simulink model "MSC_MATLAB_AGV_ROMB_diploma_3pcs_final"  (R2016b)
settings: Solver=VariableStepAuto  StartTime=0.0  StopTime=100  RelTol=1e-3
PreLoadFcn:
  | load('C:\Users\CAD_Admin\AGV\gostask\warehouse1.mat')
  | AGV_Simple_ New
values from neighbouring files (symbols this model uses):
  AGVs =     [algorithm_test.mat]
  contr1_kp = 0.4    [algorithm_test.mat]
  LF_AngVel = 30    [algorithm_test.mat]
  lns = lns1    [CMDTrackRead.m]    (also in algorithm_test.mat = [1 3 5 7 9 11 13 15 17 19 21 23 ... (242 elements, 121x2)]; warehouseGubkina.mat = [9 3 2 10 4 8 7 3 8 5 7 6 ... (26 elements, 13x2)]; warehouseGubkinaNew.mat = [9 15 17 10 19 11 13 3 3 5 5 8 ... (46 elements, 23x2)])
  pnts = RoundingPnts(pnts)    [Avoidance_Testing.m]    (also in CMDTrackRead.m = pnts1; algorithm_test.mat = [-350 450 0 0 100 100 -340 -260 -100 -100 -350 450 ... (321 ; warehouseGubkina.mat = [4100 4100 4100 3646 3646 3646 3822 3822 4100 4198.5 3822 34; warehouseGubkinaNew.mat = [4100 4100 4100 3646 3646 3646 3822 3822 4100 4198.5 3822 38)
  SteeringVel = 10    [algorithm_test.mat]
  T_Motor = 0.05    [algorithm_test.mat]
  tau_DiscreteSensor = 0.3    [algorithm_test.mat]
  tau_Motor = 0.125    [algorithm_test.mat]
  value0 = [23350 22900 22450 20300 17050 13100 10500 8700 8100 7800 7700 7800 ... (21 elements, 21x1)]    [algorithm_test.mat]
  x0 = 10    [SecondAGV.m]    (also in algorithm_test.mat = [-70 -50 -40 -35 -30 -25 -20 -15 -10 -5 0 5 ... (21 elements)
undefined symbols (not defined in the file): ADAMS_cwd, ADAMS_exec, ADAMS_host, ADAMS_init, ADAMS_inputs, ADAMS_outputs, ADAMS_prefix, ADAMS_static, ADAMS_sysdir
libraries: simulink x21
(part 2 of 2)

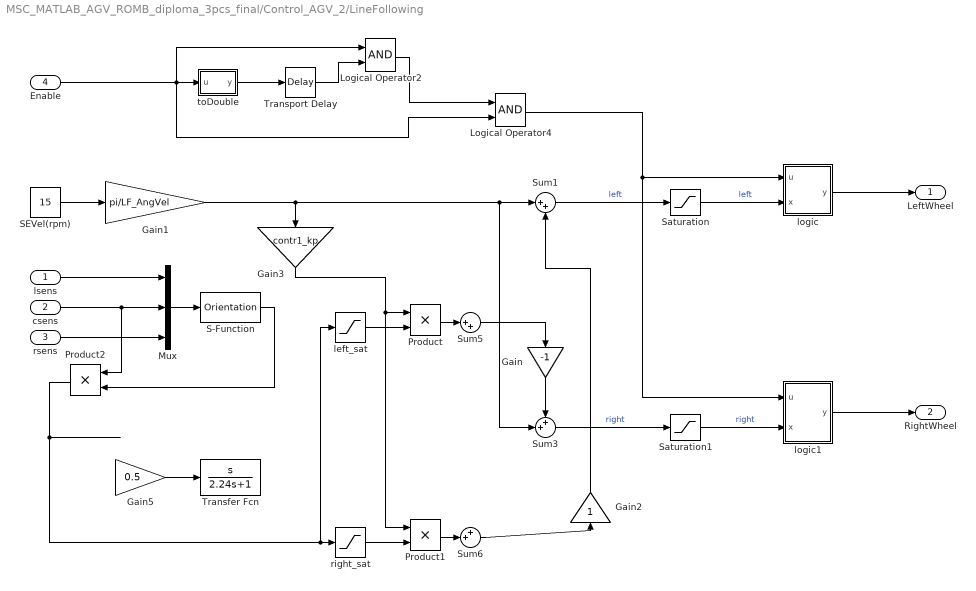
== system MSC_MATLAB_AGV_ROMB_diploma_3pcs_final/Control_AGV_2/LineFollowing ==
  lsens : Inport
  csens : Inport  Port=2
  rsens : Inport  Port=3
  Enable : Inport  Port=4
  Gain : Gain  Gain=-1
  Gain1 : Gain  Gain=pi/LF_AngVel
  Gain2 : Gain
  Gain3 : Gain  Gain=contr1_kp
  Gain5 : Gain  Gain=0.5
  Logical Operator2 : Logic  AllPortsSameDT=off  OutDataTypeStr=boolean
  Logical Operator4 : Logic  AllPortsSameDT=off  OutDataTypeStr=boolean
  Mux : Mux  Inputs=3
  Product : Product
  Product1 : Product
  Product2 : Product
  S-Function : S-Function  FunctionName=Orientation  SFunctionDeploymentMode=off  EnableBusSupport=off
  SEVel(rpm) : Constant  Value=15
  Saturation : Saturate  UpperLimit=inf  LowerLimit=0
  Saturation1 : Saturate  UpperLimit=inf  LowerLimit=0
  Sum1 : Sum  Inputs=|++
  Sum3 : Sum  Inputs=++|
  Sum5 : Sum  Inputs=|++
  Sum6 : Sum  Inputs=++|
  Transfer Fcn : TransferFcn  Numerator=[1 0]  Denominator=[2.24 1]
  Transport Delay : TransportDelay  DelayTime=0.05
  left_sat : Saturate  UpperLimit=0  LowerLimit=-10
  logic : MATLAB Function  TreatAsAtomicUnit=on
  logic1 : MATLAB Function  TreatAsAtomicUnit=on
  right_sat : Saturate  UpperLimit=10  LowerLimit=0
  toDouble : MATLAB Function  TreatAsAtomicUnit=on
  LeftWheel : Outport
  RightWheel : Outport  Port=2
  wires:
  SEVel(rpm)/1 -> Gain1/1
  Gain1/1 -> Sum3/2, Sum1/1, Gain3/1
  lsens/1 -> Mux/1
  rsens/1 -> Mux/3
  Sum6/1 -> Gain2/1
  S-Function/1 -> Product2/2
  csens/1 -> Product2/1, Mux/2
  Product2/1 -> left_sat/1, right_sat/1
  Saturation/1 -> logic/2(x)  "left"
  logic/1(y) -> LeftWheel/1
  Saturation1/1 -> logic1/2(x)  "right"
  logic1/1(y) -> RightWheel/1
  Logical Operator2/1 -> Logical Operator4/1
  Enable/1 -> Logical Operator2/1, toDouble/1(u), Logical Operator4/2
  toDouble/1(y) -> Transport Delay/1
  Transport Delay/1 -> Logical Operator2/2
  Logical Operator4/1 -> logic1/1(u), logic/1(u)
  Mux/1 -> S-Function/1
  Gain/1 -> Sum3/1
  Gain2/1 -> Sum1/2
  Sum5/1 -> Gain/1
  Gain3/1 -> Product1/1, Product/1
  right_sat/1 -> Product1/2
  left_sat/1 -> Product/2
  Gain5/1 -> Transfer Fcn/1
  ? -> Sum6/1, Sum5/2
  Product/1 -> Sum5/1
  Product1/1 -> Sum6/2
  Sum3/1 -> Saturation1/1  "right"
  Sum1/1 -> Saturation/1  "left"

== system MSC_MATLAB_AGV_ROMB_diploma_3pcs_final/Control_AGV_2/Steering ==
  lsens : Inport
  csens : Inport  Port=2
  rsens : Inport  Port=3
  Steering : Inport  Port=4
  Enable : Inport  Port=5
  Demux : Demux  Outputs=2
  Gain1 : Gain  Gain=pi/LF_AngVel
  Logical Operator2 : Logic  AllPortsSameDT=off  OutDataTypeStr=boolean
  Logical Operator4 : Logic  AllPortsSameDT=off  OutDataTypeStr=boolean
  Mux : Mux
  Product : Product
  Product2 : Product
  S-Function : S-Function  FunctionName=CartSteering_1  Parameters=lns,pnts  SFunctionDeploymentMode=off  EnableBusSupport=off
  SEVel(rpm) : Constant  Value=SteeringVel
  Saturation : Saturate  UpperLimit=inf  LowerLimit=-inf
  Saturation1 : Saturate  UpperLimit=inf  LowerLimit=-inf
  Transport Delay : TransportDelay  DelayTime=0.2
  left_sat : Saturate  UpperLimit=2  LowerLimit=-2
  logic : MATLAB Function  TreatAsAtomicUnit=on
  logic1 : MATLAB Function  TreatAsAtomicUnit=on
  right_sat : Saturate  UpperLimit=2  LowerLimit=-2
  toDouble : MATLAB Function  TreatAsAtomicUnit=on
  LeftWheel : Outport
  RightWheel : Outport  Port=2
  wires:
  rsens/1 -> Mux/3
  csens/1 -> Mux/2
  lsens/1 -> Mux/1
  Steering/1 -> Mux/4
  Product/1 -> Saturation/1  "left"
  SEVel(rpm)/1 -> Gain1/1
  Product2/1 -> Saturation1/1  "right"
  Gain1/1 -> Product2/1, Product/1
  Saturation/1 -> logic/2(x)  "left"
  Saturation1/1 -> logic1/2(x)  "right"
  Demux/1 -> left_sat/1
  Demux/2 -> right_sat/1
  Mux/1 -> S-Function/1
  S-Function/1 -> Demux/1
  left_sat/1 -> Product/2
  right_sat/1 -> Product2/2
  logic/1(y) -> LeftWheel/1
  logic1/1(y) -> RightWheel/1
  Logical Operator4/1 -> logic1/1(u), logic/1(u)
  Logical Operator2/1 -> Logical Operator4/1
  Enable/1 -> toDouble/1(u), Logical Operator4/2, Logical Operator2/1
  toDouble/1(y) -> Transport Delay/1
  Transport Delay/1 -> Logical Operator2/2

== system MSC_MATLAB_AGV_ROMB_diploma_3pcs_final/Control_AGV_2/Subsystem ==
  Enable : Inport
  LeftWheel : Inport  Port=2
  RightWheel : Inport  Port=3
  Logical Operator2 : Logic  AllPortsSameDT=off  OutDataTypeStr=boolean
  Logical Operator4 : Logic  AllPortsSameDT=off  OutDataTypeStr=boolean
  Transport Delay1 : TransportDelay  DelayTime=0.05
  logic : MATLAB Function  TreatAsAtomicUnit=on
  logic1 : MATLAB Function  TreatAsAtomicUnit=on
  toDouble5 : MATLAB Function  TreatAsAtomicUnit=on
  LeftVel : Outport
  RightVel : Outport  Port=2
  wires:
  Logical Operator2/1 -> Logical Operator4/1
  Enable/1 -> Logical Operator2/1, toDouble5/1(u), Logical Operator4/2
  toDouble5/1(y) -> Transport Delay1/1
  Transport Delay1/1 -> Logical Operator2/2
  Logical Operator4/1 -> logic1/1(u), logic/1(u)
  logic/1(y) -> LeftVel/1
  logic1/1(y) -> RightVel/1
  LeftWheel/1 -> logic/2(x)
  RightWheel/1 -> logic1/2(x)

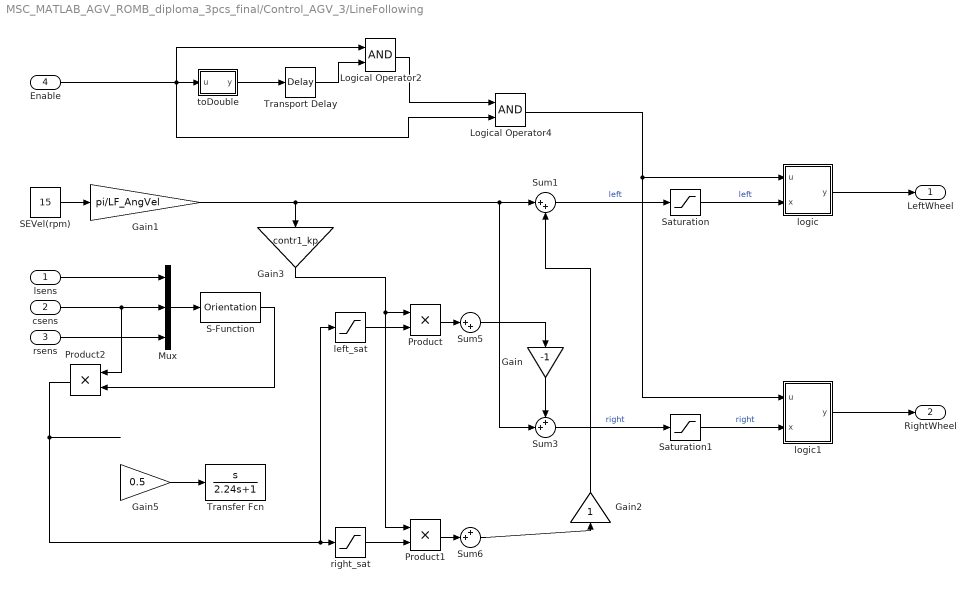
== system MSC_MATLAB_AGV_ROMB_diploma_3pcs_final/Control_AGV_3/LineFollowing ==
  lsens : Inport
  csens : Inport  Port=2
  rsens : Inport  Port=3
  Enable : Inport  Port=4
  Gain : Gain  Gain=-1
  Gain1 : Gain  Gain=pi/LF_AngVel
  Gain2 : Gain
  Gain3 : Gain  Gain=contr1_kp
  Gain5 : Gain  Gain=0.5
  Logical Operator2 : Logic  AllPortsSameDT=off  OutDataTypeStr=boolean
  Logical Operator4 : Logic  AllPortsSameDT=off  OutDataTypeStr=boolean
  Mux : Mux  Inputs=3
  Product : Product
  Product1 : Product
  Product2 : Product
  S-Function : S-Function  FunctionName=Orientation  SFunctionDeploymentMode=off  EnableBusSupport=off
  SEVel(rpm) : Constant  Value=15
  Saturation : Saturate  UpperLimit=inf  LowerLimit=0
  Saturation1 : Saturate  UpperLimit=inf  LowerLimit=0
  Sum1 : Sum  Inputs=|++
  Sum3 : Sum  Inputs=++|
  Sum5 : Sum  Inputs=|++
  Sum6 : Sum  Inputs=++|
  Transfer Fcn : TransferFcn  Numerator=[1 0]  Denominator=[2.24 1]
  Transport Delay : TransportDelay  DelayTime=0.05
  left_sat : Saturate  UpperLimit=0  LowerLimit=-10
  logic : MATLAB Function  TreatAsAtomicUnit=on
  logic1 : MATLAB Function  TreatAsAtomicUnit=on
  right_sat : Saturate  UpperLimit=10  LowerLimit=0
  toDouble : MATLAB Function  TreatAsAtomicUnit=on
  LeftWheel : Outport
  RightWheel : Outport  Port=2
  wires:
  SEVel(rpm)/1 -> Gain1/1
  Gain1/1 -> Sum3/2, Sum1/1, Gain3/1
  lsens/1 -> Mux/1
  rsens/1 -> Mux/3
  Sum6/1 -> Gain2/1
  S-Function/1 -> Product2/2
  csens/1 -> Product2/1, Mux/2
  Product2/1 -> left_sat/1, right_sat/1
  Saturation/1 -> logic/2(x)  "left"
  logic/1(y) -> LeftWheel/1
  Saturation1/1 -> logic1/2(x)  "right"
  logic1/1(y) -> RightWheel/1
  Logical Operator2/1 -> Logical Operator4/1
  Enable/1 -> Logical Operator2/1, toDouble/1(u), Logical Operator4/2
  toDouble/1(y) -> Transport Delay/1
  Transport Delay/1 -> Logical Operator2/2
  Logical Operator4/1 -> logic1/1(u), logic/1(u)
  Mux/1 -> S-Function/1
  Gain/1 -> Sum3/1
  Gain2/1 -> Sum1/2
  Sum5/1 -> Gain/1
  Gain3/1 -> Product1/1, Product/1
  right_sat/1 -> Product1/2
  left_sat/1 -> Product/2
  Gain5/1 -> Transfer Fcn/1
  ? -> Sum6/1, Sum5/2
  Product/1 -> Sum5/1
  Product1/1 -> Sum6/2
  Sum3/1 -> Saturation1/1  "right"
  Sum1/1 -> Saturation/1  "left"

== system MSC_MATLAB_AGV_ROMB_diploma_3pcs_final/Control_AGV_3/Steering ==
  lsens : Inport
  csens : Inport  Port=2
  rsens : Inport  Port=3
  Steering : Inport  Port=4
  Enable : Inport  Port=5
  Demux : Demux  Outputs=2
  Gain1 : Gain  Gain=pi/LF_AngVel
  Logical Operator2 : Logic  AllPortsSameDT=off  OutDataTypeStr=boolean
  Logical Operator4 : Logic  AllPortsSameDT=off  OutDataTypeStr=boolean
  Mux : Mux
  Product : Product
  Product2 : Product
  S-Function : S-Function  FunctionName=CartSteering_1  Parameters=lns,pnts  SFunctionDeploymentMode=off  EnableBusSupport=off
  SEVel(rpm) : Constant  Value=SteeringVel
  Saturation : Saturate  UpperLimit=inf  LowerLimit=-inf
  Saturation1 : Saturate  UpperLimit=inf  LowerLimit=-inf
  Transport Delay : TransportDelay  DelayTime=0.2
  left_sat : Saturate  UpperLimit=2  LowerLimit=-2
  logic : MATLAB Function  TreatAsAtomicUnit=on
  logic1 : MATLAB Function  TreatAsAtomicUnit=on
  right_sat : Saturate  UpperLimit=2  LowerLimit=-2
  toDouble : MATLAB Function  TreatAsAtomicUnit=on
  LeftWheel : Outport
  RightWheel : Outport  Port=2
  wires:
  rsens/1 -> Mux/3
  csens/1 -> Mux/2
  lsens/1 -> Mux/1
  Steering/1 -> Mux/4
  Product/1 -> Saturation/1  "left"
  SEVel(rpm)/1 -> Gain1/1
  Product2/1 -> Saturation1/1  "right"
  Gain1/1 -> Product2/1, Product/1
  Saturation/1 -> logic/2(x)  "left"
  Saturation1/1 -> logic1/2(x)  "right"
  Demux/1 -> left_sat/1
  Demux/2 -> right_sat/1
  Mux/1 -> S-Function/1
  S-Function/1 -> Demux/1
  left_sat/1 -> Product/2
  right_sat/1 -> Product2/2
  logic/1(y) -> LeftWheel/1
  logic1/1(y) -> RightWheel/1
  Logical Operator4/1 -> logic1/1(u), logic/1(u)
  Logical Operator2/1 -> Logical Operator4/1
  Enable/1 -> toDouble/1(u), Logical Operator4/2, Logical Operator2/1
  toDouble/1(y) -> Transport Delay/1
  Transport Delay/1 -> Logical Operator2/2

== system MSC_MATLAB_AGV_ROMB_diploma_3pcs_final/Control_AGV_3/Subsystem ==
  Enable : Inport
  LeftWheel : Inport  Port=2
  RightWheel : Inport  Port=3
  Logical Operator2 : Logic  AllPortsSameDT=off  OutDataTypeStr=boolean
  Logical Operator4 : Logic  AllPortsSameDT=off  OutDataTypeStr=boolean
  Transport Delay1 : TransportDelay  DelayTime=0.05
  logic : MATLAB Function  TreatAsAtomicUnit=on
  logic1 : MATLAB Function  TreatAsAtomicUnit=on
  toDouble5 : MATLAB Function  TreatAsAtomicUnit=on
  LeftVel : Outport
  RightVel : Outport  Port=2
  wires:
  Logical Operator2/1 -> Logical Operator4/1
  Enable/1 -> Logical Operator2/1, toDouble5/1(u), Logical Operator4/2
  toDouble5/1(y) -> Transport Delay1/1
  Transport Delay1/1 -> Logical Operator2/2
  Logical Operator4/1 -> logic1/1(u), logic/1(u)
  logic/1(y) -> LeftVel/1
  logic1/1(y) -> RightVel/1
  LeftWheel/1 -> logic/2(x)
  RightWheel/1 -> logic1/2(x)

== system MSC_MATLAB_AGV_ROMB_diploma_3pcs_final/adams_sub/ADAMS Plant ==
  ADAMS inputs : Inport
  S-Function : S-Function  StopFcn=clear mex  FunctionName=adams_plant  Parameters=exevie,exesol,stat,outfil,nampre,o_rate,nam_in,namout,dft,modsim,modani,dt_out,inicmd,exetyp,comtyp,ada_host, workdir,pin_interp_order,pout_extrap_order,pin_extrap_order,pout_interp_order,simulink_lead_cosim  SFunctionDeploymentMode=off  EnableBusSupport=off
  ADAMS outputs : Outport  InitialOutput=0
  wires:
  ADAMS inputs/1 -> S-Function/1
  S-Function/1 -> ADAMS outputs/1

== matlab function MSC_MATLAB_AGV_ROMB_diploma_3pcs_final/Sensors_AGV_1/Sensors ==
  data: lx input; ldist output; ly input; cx input; cy input; rx input; ry input; rfx input; rfy input; lns input; pnts input; cdist output; rdist output; lsens output; csens output; rsens output; numrfid output; dst output; x0 input; value0 input
function [ldist, cdist, rdist, lsens, csens, rsens, numrfid, dst] = fcn(lx, ly, cx, cy, rx, ry, rfx, rfy, lns, pnts, x0, value0)

p00 = [0 0 0]; % p00 = [4100 0 -2196];          % Center of coordinates (Matlab)

lpoint = [lx ly 0] + p00;      % Coordinate of left sensor (Adams to Matlab)  
cpoint = [cx cy 0] + p00;      % Coordinate of center sensor (Adams to Matlab)  
rpoint = [rx ry 0] + p00;      % Coordinate of right sensor (Adams to Matlab)  
rfpoint = [rfx rfy 0] + p00;   % Coordinate of RFID reader (Adams to Matlab) rfy - 50

ldist = min(DistanceLinePoint(pnts,lns,lpoint));
cdist = min(DistanceLinePoint(pnts,lns,cpoint));
rdist = min(DistanceLinePoint(pnts,lns,rpoint));

if (ldist >= 3) 
    lsens = 0;
else
    lsens = 1;
end;

if (rdist >= 3) 
    rsens = 0;
else
    rsens = 1;
end;

%if (cdist >= 5.81) 
  %  csens = 5.81;
%else
  %  csens=cdist;
%end;
% csens = 2.8801 - 1.266 * exp( - ( ( cdist * 10 ) ^ 2 / 612.0676 ) ) - 1.5;
csens = ((interp1(x0,value0, cdist * 10,'linear',23350) - min(value0)) / 32767 ) * 4.096 + 0.05;

% if csens < 0 
%     Psy = 1;
% end

%numrfid=0;
[dst,numrfid] = min(DistancePointPoint(pnts,rfpoint));
if (dst > 3) % before 15ss % after 45
    numrfid = 0;
end;

== matlab function MSC_MATLAB_AGV_ROMB_diploma_3pcs_final/Sensors_AGV_2/Sensors ==
  data: lx input; ldist output; ly input; cx input; cy input; rx input; ry input; rfx input; rfy input; lns input; pnts input; cdist output; rdist output; lsens output; csens output; rsens output; numrfid output; dst output; x0 input; value0 input
function [ldist, cdist, rdist, lsens, csens, rsens, numrfid, dst] = fcn(lx, ly, cx, cy, rx, ry, rfx, rfy, lns, pnts, x0, value0)

p00 = [0 0 0]; % p00 = [4100 0 -2196];          % Center of coordinates (Matlab)

lpoint = [lx ly 0] + p00;      % Coordinate of left sensor (Adams to Matlab)  
cpoint = [cx cy 0] + p00;      % Coordinate of center sensor (Adams to Matlab)  
rpoint = [rx ry 0] + p00;      % Coordinate of right sensor (Adams to Matlab)  
rfpoint = [rfx rfy 0] + p00;   % Coordinate of RFID reader (Adams to Matlab) rfy - 50

ldist = min(DistanceLinePoint(pnts,lns,lpoint));
cdist = min(DistanceLinePoint(pnts,lns,cpoint));
rdist = min(DistanceLinePoint(pnts,lns,rpoint));

if (ldist >= 3) 
    lsens = 0;
else
    lsens = 1;
end;

if (rdist >= 3) 
    rsens = 0;
else
    rsens = 1;
end;

%if (cdist >= 5.81) 
  %  csens = 5.81;
%else
  %  csens=cdist;
%end;
% csens = 2.8801 - 1.266 * exp( - ( ( cdist * 10 ) ^ 2 / 612.0676 ) ) - 1.5;
csens = ((interp1(x0,value0, cdist * 10,'linear',23350) - min(value0)) / 32767 ) * 4.096 + 0.05;

% if csens < 0 
%     Psy = 1;
% end

%numrfid=0;
[dst,numrfid] = min(DistancePointPoint(pnts,rfpoint));
if (dst > 3) % before 15ss % after 45
    numrfid = 0;
end;

== matlab function MSC_MATLAB_AGV_ROMB_diploma_3pcs_final/Sensors_AGV_3/Sensors ==
  data: lx input; ldist output; ly input; cx input; cy input; rx input; ry input; rfx input; rfy input; lns input; pnts input; cdist output; rdist output; lsens output; csens output; rsens output; numrfid output; dst output; x0 input; value0 input
function [ldist, cdist, rdist, lsens, csens, rsens, numrfid, dst] = fcn(lx, ly, cx, cy, rx, ry, rfx, rfy, lns, pnts, x0, value0)

p00 = [0 0 0]; % p00 = [4100 0 -2196];          % Center of coordinates (Matlab)

lpoint = [lx ly 0] + p00;      % Coordinate of left sensor (Adams to Matlab)  
cpoint = [cx cy 0] + p00;      % Coordinate of center sensor (Adams to Matlab)  
rpoint = [rx ry 0] + p00;      % Coordinate of right sensor (Adams to Matlab)  
rfpoint = [rfx rfy 0] + p00;   % Coordinate of RFID reader (Adams to Matlab) rfy - 50

ldist = min(DistanceLinePoint(pnts,lns,lpoint));
cdist = min(DistanceLinePoint(pnts,lns,cpoint));
rdist = min(DistanceLinePoint(pnts,lns,rpoint));

if (ldist >= 3) 
    lsens = 0;
else
    lsens = 1;
end;

if (rdist >= 3) 
    rsens = 0;
else
    rsens = 1;
end;

%if (cdist >= 5.81) 
  %  csens = 5.81;
%else
  %  csens=cdist;
%end;
% csens = 2.8801 - 1.266 * exp( - ( ( cdist * 10 ) ^ 2 / 612.0676 ) ) - 1.5;
csens = ((interp1(x0,value0, cdist * 10,'linear',23350) - min(value0)) / 32767 ) * 4.096 + 0.05;

% if csens < 0 
%     Psy = 1;
% end

%numrfid=0;
[dst,numrfid] = min(DistancePointPoint(pnts,rfpoint));
if (dst > 3) % before 15ss % after 45
    numrfid = 0;
end;

== matlab function MSC_MATLAB_AGV_ROMB_diploma_3pcs_final/Control_AGV_2/LineFollowing/logic ==
  data: u input; y output; x input
function y = fcn(u, x)
if (u == true)
    y = x;
else
    y = 0;
end;

== matlab function MSC_MATLAB_AGV_ROMB_diploma_3pcs_final/Control_AGV_2/LineFollowing/logic1 ==
  data: u input; y output; x input
function y = fcn(u, x)
if (u == true)
    y = x;
else
    y = 0;
end;

== matlab function MSC_MATLAB_AGV_ROMB_diploma_3pcs_final/Control_AGV_2/LineFollowing/toDouble ==
  data: u input; y output
function y = fcn(u)

y = double(u);

== matlab function MSC_MATLAB_AGV_ROMB_diploma_3pcs_final/Control_AGV_2/Steering/logic ==
  data: u input; y output; x input
function y = fcn(u, x)
if (u == true)
    y = x;
else
    y = 0;
end;

== matlab function MSC_MATLAB_AGV_ROMB_diploma_3pcs_final/Control_AGV_2/Steering/logic1 ==
  data: u input; y output; x input
function y = fcn(u, x)
if (u == true)
    y = x;
else
    y = 0;
end;

== matlab function MSC_MATLAB_AGV_ROMB_diploma_3pcs_final/Control_AGV_2/Steering/toDouble ==
  data: u input; y output
function y = fcn(u)

y = double(u);

== matlab function MSC_MATLAB_AGV_ROMB_diploma_3pcs_final/Control_AGV_2/toDouble ==
  data: u input; y output
function y = fcn(u)

y = double(u);

== matlab function MSC_MATLAB_AGV_ROMB_diploma_3pcs_final/Control_AGV_2/toDouble1 ==
  data: u input; y output
function y = fcn(u)

y = double(u);

== matlab function MSC_MATLAB_AGV_ROMB_diploma_3pcs_final/Control_AGV_2/toDouble2 ==
  data: u input; y output
function y = fcn(u)

y = double(u);

== matlab function MSC_MATLAB_AGV_ROMB_diploma_3pcs_final/Control_AGV_1/LineFollowing/logic ==
  data: u input; y output; x input
function y = fcn(u, x)
if (u == true)
    y = x;
else
    y = 0;
end;

== matlab function MSC_MATLAB_AGV_ROMB_diploma_3pcs_final/Control_AGV_1/LineFollowing/logic1 ==
  data: u input; y output; x input
function y = fcn(u, x)
if (u == true)
    y = x;
else
    y = 0;
end;

== matlab function MSC_MATLAB_AGV_ROMB_diploma_3pcs_final/Control_AGV_1/LineFollowing/toDouble ==
  data: u input; y output
function y = fcn(u)

y = double(u);

== matlab function MSC_MATLAB_AGV_ROMB_diploma_3pcs_final/Control_AGV_1/Steering/logic ==
  data: u input; y output; x input
function y = fcn(u, x)
if (u == true)
    y = x;
else
    y = 0;
end;

== matlab function MSC_MATLAB_AGV_ROMB_diploma_3pcs_final/Control_AGV_1/Steering/logic1 ==
  data: u input; y output; x input
function y = fcn(u, x)
if (u == true)
    y = x;
else
    y = 0;
end;

== matlab function MSC_MATLAB_AGV_ROMB_diploma_3pcs_final/Control_AGV_1/Steering/toDouble ==
  data: u input; y output
function y = fcn(u)

y = double(u);

== matlab function MSC_MATLAB_AGV_ROMB_diploma_3pcs_final/Control_AGV_1/toDouble ==
  data: u input; y output
function y = fcn(u)

y = double(u);

== matlab function MSC_MATLAB_AGV_ROMB_diploma_3pcs_final/Control_AGV_1/toDouble1 ==
  data: u input; y output
function y = fcn(u)

y = double(u);

== matlab function MSC_MATLAB_AGV_ROMB_diploma_3pcs_final/Control_AGV_1/toDouble2 ==
  data: u input; y output
function y = fcn(u)

y = double(u);

== matlab function MSC_MATLAB_AGV_ROMB_diploma_3pcs_final/Control_AGV_1/toDouble3 ==
  data: u input; y output
function y = fcn(u)

y = double(u);

== matlab function MSC_MATLAB_AGV_ROMB_diploma_3pcs_final/Control_AGV_1/toDouble4 ==
  data: u input; y output
function y = fcn(u)

y = double(u);

== matlab function MSC_MATLAB_AGV_ROMB_diploma_3pcs_final/Control_AGV_2/toDouble3 ==
  data: u input; y output
function y = fcn(u)

y = double(u);

== matlab function MSC_MATLAB_AGV_ROMB_diploma_3pcs_final/Control_AGV_2/toDouble4 ==
  data: u input; y output
function y = fcn(u)

y = double(u);

== matlab function MSC_MATLAB_AGV_ROMB_diploma_3pcs_final/Control_AGV_3/LineFollowing/logic ==
  data: u input; y output; x input
function y = fcn(u, x)
if (u == true)
    y = x;
else
    y = 0;
end;

== matlab function MSC_MATLAB_AGV_ROMB_diploma_3pcs_final/Control_AGV_3/LineFollowing/logic1 ==
  data: u input; y output; x input
function y = fcn(u, x)
if (u == true)
    y = x;
else
    y = 0;
end;

== matlab function MSC_MATLAB_AGV_ROMB_diploma_3pcs_final/Control_AGV_3/LineFollowing/toDouble ==
  data: u input; y output
function y = fcn(u)

y = double(u);

== matlab function MSC_MATLAB_AGV_ROMB_diploma_3pcs_final/Control_AGV_3/Steering/logic ==
  data: u input; y output; x input
function y = fcn(u, x)
if (u == true)
    y = x;
else
    y = 0;
end;

== matlab function MSC_MATLAB_AGV_ROMB_diploma_3pcs_final/Control_AGV_3/Steering/logic1 ==
  data: u input; y output; x input
function y = fcn(u, x)
if (u == true)
    y = x;
else
    y = 0;
end;

== matlab function MSC_MATLAB_AGV_ROMB_diploma_3pcs_final/Control_AGV_3/Steering/toDouble ==
  data: u input; y output
function y = fcn(u)

y = double(u);

== matlab function MSC_MATLAB_AGV_ROMB_diploma_3pcs_final/Control_AGV_3/toDouble ==
  data: u input; y output
function y = fcn(u)

y = double(u);

== matlab function MSC_MATLAB_AGV_ROMB_diploma_3pcs_final/Control_AGV_3/toDouble1 ==
  data: u input; y output
function y = fcn(u)

y = double(u);

== matlab function MSC_MATLAB_AGV_ROMB_diploma_3pcs_final/Control_AGV_3/toDouble2 ==
  data: u input; y output
function y = fcn(u)

y = double(u);

== matlab function MSC_MATLAB_AGV_ROMB_diploma_3pcs_final/Control_AGV_3/toDouble3 ==
  data: u input; y output
function y = fcn(u)

y = double(u);

== matlab function MSC_MATLAB_AGV_ROMB_diploma_3pcs_final/Control_AGV_3/toDouble4 ==
  data: u input; y output
function y = fcn(u)

y = double(u);

== matlab function MSC_MATLAB_AGV_ROMB_diploma_3pcs_final/Control_AGV_1/Actuator_Control ==
  data: u input; y output; numrfid input; StopWheel output
function [y, StopWheel] = fcn(u, numrfid)

if numrfid == 1 || numrfid == 93
    Actuator = 1; % Lift
elseif numrfid == 1 || numrfid == 10
    Actuator = 2; % Drop
else
    Actuator = 0; % Nothing
end;

if (u < 25) && (Actuator == 1)
    y = 0.75;
    StopWheel = false;
elseif (u > 12) && (Actuator == 2)
    y = -0.75;
    StopWheel = false;
else
    y = 0;
    StopWheel = true;
end;

end

== matlab function MSC_MATLAB_AGV_ROMB_diploma_3pcs_final/Control_AGV_1/Subsystem/logic ==
  data: u input; y output; x input
function y = fcn(u, x)
if (u == true)
    y = x;
else
    y = 0;
end;

== matlab function MSC_MATLAB_AGV_ROMB_diploma_3pcs_final/Control_AGV_1/Subsystem/logic1 ==
  data: u input; y output; x input
function y = fcn(u, x)
if (u == true)
    y = x;
else
    y = 0;
end;

== matlab function MSC_MATLAB_AGV_ROMB_diploma_3pcs_final/Control_AGV_1/Subsystem/toDouble5 ==
  data: u input; y output
function y = fcn(u)

y = double(u);

== matlab function MSC_MATLAB_AGV_ROMB_diploma_3pcs_final/Control_AGV_2/Actuator_Control_2 ==
  data: u input; y output; numrfid input; StopWheel output
function [y, StopWheel] = fcn(u, numrfid)

if numrfid == 1 || numrfid == 10
    Actuator = 1; % Lift
elseif numrfid == 1 || numrfid == 10
    Actuator = 2; % Drop
else
    Actuator = 0; % Nothing
end;

if (u < 25) && (Actuator == 1)
    y = 0.5;
    StopWheel = false;
elseif (u > 12) && (Actuator == 2)
    y = -0.5;
    StopWheel = false;
else
    y = 0;
    StopWheel = true;
end;

end

== matlab function MSC_MATLAB_AGV_ROMB_diploma_3pcs_final/Control_AGV_2/Subsystem/logic ==
  data: u input; y output; x input
function y = fcn(u, x)
if (u == true)
    y = x;
else
    y = 0;
end;

== matlab function MSC_MATLAB_AGV_ROMB_diploma_3pcs_final/Control_AGV_2/Subsystem/logic1 ==
  data: u input; y output; x input
function y = fcn(u, x)
if (u == true)
    y = x;
else
    y = 0;
end;

== matlab function MSC_MATLAB_AGV_ROMB_diploma_3pcs_final/Control_AGV_2/Subsystem/toDouble5 ==
  data: u input; y output
function y = fcn(u)

y = double(u);

== matlab function MSC_MATLAB_AGV_ROMB_diploma_3pcs_final/Control_AGV_3/Actuator_Control_3 ==
  data: u input; y output; numrfid input; StopWheel output
function [y, StopWheel] = fcn(u, numrfid)

if numrfid == 79 || numrfid == 10
    Actuator = 1; % Lift
elseif numrfid == 80 || numrfid == 10
    Actuator = 2; % Drop
else
    Actuator = 0; % Nothing
end;

if (u < 25) && (Actuator == 1)
    y = 0.5;
    StopWheel = false;
elseif (u > 12) && (Actuator == 2)
    y = -0.5;
    StopWheel = false;
else
    y = 0;
    StopWheel = true;
end;

end

== matlab function MSC_MATLAB_AGV_ROMB_diploma_3pcs_final/Control_AGV_3/Subsystem/logic ==
  data: u input; y output; x input
function y = fcn(u, x)
if (u == true)
    y = x;
else
    y = 0;
end;

== matlab function MSC_MATLAB_AGV_ROMB_diploma_3pcs_final/Control_AGV_3/Subsystem/logic1 ==
  data: u input; y output; x input
function y = fcn(u, x)
if (u == true)
    y = x;
else
    y = 0;
end;

== matlab function MSC_MATLAB_AGV_ROMB_diploma_3pcs_final/Control_AGV_3/Subsystem/toDouble5 ==
  data: u input; y output
function y = fcn(u)

y = double(u);
